simulink model "SmallFixedWingUAVupperHIL"  (R2022b)
settings: Solver=FixedStepDiscrete  StartTime=0.0  StopTime=inf  FixedStep=1/300  RelTol=1e-3
model workspace: external: MAT-File E:\RFLY\small-fixed-wing-book\fixedwing-book-rfly\ch8\code\e7-4\hitl\desire.mat (data not in the file)
values from neighbouring files (symbols this model uses):
  ctrlpoints = [xd'-xd(1);yd'-yd(1)]    [bspline.m]
  env = struct    [InitDatactrl.m]
  knots = [t1, t2, t3]    [bspline.m]
  pp = 3    [bspline.m]
  uav = struct    [InitDatactrl.m]
undefined symbols (not defined in the file or in its folder): DiscIntNeverNeededParam, RGBLED_COLOR_ENUM, RGBLED_MODE_ENUM
libraries: simulink x10, pixhawk_slib_sensors_actuators x6, pixhawk_slib_uORB_RW x5
(part 2 of 2)

== matlab function SmallFixedWingUAVupperHIL/Command/MATLAB Function8 ==
  data: n input; C output; t input; P input; U input
function C = bspline_deboor(n,t,P,U)
%     validateattributes(n, {'numeric'}, {'positive','integer','scalar'});
    d = n;  % B-spline polynomial degree (1 for linear, 2 for quadratic, etc.)
%     validateattributes(t, {'numeric'}, {'real','vector'});
%     assert(all( t(2:end)-t(1:end-1) >= 0 ), 'bspline:deboor:InvalidArgumentValue', ...
%         'Knot vector values should be nondecreasing.');
%     validateattributes(P, {'numeric'}, {'real','2d'});
%     
%     if nargin < 4
%         U = linspace(t(d+1), t(end-d), 10*size(P,2));  % allocate points uniformly
%     elseif isscalar(U) && U > 1
%         validateattributes(U, {'numeric'}, {'positive','integer','scalar'});
%         U = linspace(t(d+1), t(end-d), U);  % allocate points uniformly
%     else
%         validateattributes(U, {'numeric'}, {'real','vector'});
%         assert(all( U >= t(d+1) & U <= t(end-d) ), 'bspline:deboor:InvalidArgumentValue', ...
%             'Value outside permitted knot vector value range.');
%     end
    
    m = size(P,1);  % dimension of control points
    t = t(:).';     % knot sequence
    U = U(:);
    S = sum(bsxfun(@eq, U, t), 2);  % multiplicity of u in t (0 <= s <= d+1)
    I = bspline_deboor_interval(U,t);
    if I>length(t)-d-1
       I=length(t)-d-1;
    end
    if I == -1
        I = length(t)-d-1;
    end
    Pk = zeros(m,d+40,d+40);
    a = zeros(d+40,d+40);
    
    C = zeros(size(P,1), numel(U));
    for j = 1 : numel(U)
        u = U(j);
        s = S(j);
        ix = I(j);
        Pk(:) = 0;
        a(:) = 0;
    
        % identify d+1 relevant control points
%         Pk(:, (ix-d):(ix-s), 1) = P(:, (ix-d):(ix-s));
        h = d - s;
        if h > 0 
            Pk(:, (ix-d):(ix-s), 1) = P(:, (ix-d):(ix-s));
        end
        if h > 0
            % de Boor recursion formula
            for r = 1 : h
                q = ix-1;
                for i = (q-d+r) : (q-s)
                    a(i+1,r+1) = (u-t(i+1)) / (t(i+d-r+1+1)-t(i+1));
                    Pk(:,i+1,r+1) = (1-a(i+1,r+1)) * Pk(:,i,r) + a(i+1,r+1) * Pk(:,i+1,r);
                end
            end
            C(:,j) = Pk(:,ix-s,d-s+1);  % extract value from triangular computation scheme
        elseif ix == numel(t)  % last control point is a special case
            C(:,j) = P(:,end);
        else
            C(:,j) = P(:,ix-d);
        end
    end
end

function ix = bspline_deboor_interval(u,t)
% Index of knot in knot sequence not less than the value of u.
% If knot has multiplicity greater than 1, the highest index is returned.
    for i = 1:length(t)
        if t(i)>u
            ix = i;
            return
        end
    end
    ix = -1;
end

% function ix = bspline_deboor_interval(u,t)
% % Index of knot in knot sequence not less than the value of u.
% % If knot has multiplicity greater than 1, the highest index is returned.
% 
% i = bsxfun(@ge, u, t) & bsxfun(@lt, u, [t(2:end) 2*t(end)]);  % indicator of knot interval in which u is
% [row,col] = find(i);
% [row,ind] = sort(row);  % restore original order of data points
% ix = col(ind);
% end

== matlab function SmallFixedWingUAVupperHIL/Command/MATLAB Function9 ==
  data: p output; order input; dknots output; knots input; ctrl input; dctrl output
function [p, dknots, dctrl] = bspline_deriv(order, knots, ctrl)
    p = order;
    tmp = size(ctrl);
    n = tmp(2)-1;
    dim = tmp(1);
    
    % derivative knots
    dknots = knots(2:max(size(knots))-1);
    
    % derivative control points
    dctrl = zeros(dim,n);
    for i = 1 : n
        dctrl(:,i) = (p / (knots(i+p+1) - knots(i+1))) * (ctrl(:,i+1) - ctrl(:,i));
    end
    p = order-1;
end

== matlab function SmallFixedWingUAVupperHIL/Command/MATLAB Function ==
  data: yaw input size=[1,1]; yawdes input; roll output size=[1,1]; g input size=[1,1]; V input size=[1,1]; rolldes input
function roll = fcn(yaw,yawdes,g,V,rolldes)
%     roll = yawrate*g*V;
    if yaw>pi
        yaw = yaw-2*pi;
    end
    yawrate = 2*(yawdes-yaw);
    roll = atan2(V.*yawrate,g);
end

== matlab function SmallFixedWingUAVupperHIL/Command/MATLAB Function3 ==
  data: av1 output; Hz output; xd input; dxd input; ddxd input; x input; dx input; yaw output; g input; roll output
function [av1,Hz,yaw,roll] = DF(xd,dxd,ddxd,x,dx,g)
    av1 = (0); 
    Hz= (0); 
    yaw= (0); 
    roll= (0); 
    xd = [xd(1);xd(2);xd(3)];
    dxd = [dxd(1);dxd(2);dxd(3)];
    ddxd = [ddxd(1);ddxd(2);ddxd(3)];
    x = [x(1);x(2);x(3)];
    dx = [dx(1);dx(2);dx(3)];
%     x1 = (xd-x)/norm(xd-x);
    r1 = zeros(3,1);
    r1 = (dxd+0.2*(xd-x))/(norm(dxd+0.2*(xd-x))+0.001);
    


    av1 = ( r1'*(1*ddxd-[0;0;g]+5*(dxd-dx)+3*(xd-x)));
     %%
%     t1 = zeros(3,1,'single');
%     t2 = zeros(3,1,'single');
%     t3 = zeros(3,1,'single');
%     t4 = zeros(3,1,'single');
%     t1(1,1) = ddxd(1,1);
%     t1(2,1) = ddxd(2,1);
%     t1(3,1) = ddxd(3,1) - single(g);
%     
%     for i = 1:3
%     t2(i,1) = single(3) * (dxd(i,1) - dx(i,1));
%     t3(i,1) = single(0.1) * (xd(i,1) - x(i,1));
% 
%     end
% 
%     for i = 1:3
%     t4(i,1) = t1(i,1) + t2(i,1) + t3(i,1);
%     end
%     av1 = single( r1'*t4);
%%

    an = (eye(3)-(r1*r1'))*((ddxd)-([0;0;g]));

    av3 = -(norm(an));
    
    Hz = (xd(3));


    r3 = (an)/((av3)+(0.001));

    r2 = cross(r3,r1);

    yaw = (atan2(r1(2),r1(1)));
    
    roll = (atan2(r2(3),r3(3)));

    if isnan(av1)
        av1=(0);
    end
    if isnan(Hz)
        Hz=(0);
    end
    if isnan(yaw)
        yaw=(0);
    end

end

== matlab function SmallFixedWingUAVupperHIL/Command/InputConditioning/deadzone0 ==
  data: u input; y output
function y = fcn(u)
%Function description:
%  Control the range of the remote control input from RCMin to RCMax,which can be obtained from QGC. And set
%  a dead zone with a dead zone size of deadZone,the output y is normalized to 0~1.
RCMin = 1100;
RCMax = 1900;
RCMid = (RCMin + RCMax)/2;
deadZoneRate = 0.05;
deadZone = deadZoneRate*(RCMax - RCMin);
k = 1/(RCMax - RCMid - deadZone);
%Limiting
if(u < RCMin)
    u = RCMin;
elseif(u > RCMax)
    u = RCMax;
end
%dead zone and normalize
 if(u > RCMid + deadZone)
    y = (u-RCMid - deadZone)*k;
 elseif(u < RCMid - deadZone)
     y = (u - RCMid + deadZone)*k;
 else
     y = 0;
 end

 end

== matlab function SmallFixedWingUAVupperHIL/Command/InputConditioning/deadzone1 ==
  data: u input; y output
function y = fcn(u)
%Function description:
%  Control the range of the remote control input from RCMin to RCMax, and set
%  a dead zone with a dead zone size of ±deadZone,the output y is
%  normalized to 0~1.You can get the RC calibration parameters in QGC.
RCMin = 1100;
RCMax = 1900;
RCMid = (RCMin + RCMax)/2;
deadZoneRate = 0.05;
deadZone = deadZoneRate*(RCMax - RCMin);
k = 1/(RCMax - RCMid - deadZone);
%Limiting
if(u < RCMin)
    u = RCMin;
elseif(u > RCMax)
    u = RCMax;
end
%dead zone and normalize
 if(u > RCMid + deadZone)
    y = (u-RCMid - deadZone)*k;
 elseif(u < RCMid - deadZone)
     y = (u - RCMid + deadZone)*k;
 else
     y = 0;
 end

 end

== matlab function SmallFixedWingUAVupperHIL/Command/InputConditioning/deadzone2 ==
  data: u input; y output
function y = fcn(u)
%Function description:
%  Control the range of the remote control input from RCMin to RCMax, and set
%  a dead zone with a dead zone size of ±deadZone,the output y is
%  normalized to 0~1.You can get the RC calibration parameters in QGC.
RCMin = 1100;
RCMax = 1900;
RCMid = (RCMin + RCMax)/2;
deadZoneRate = 0.05;
deadZone = deadZoneRate*(RCMax - RCMin);
k = 1/(RCMax - RCMid - deadZone);
%Limiting
if(u < RCMin)
    u = RCMin;
elseif(u > RCMax)
    u = RCMax;
end
%dead zone and normalize
 if(u > RCMid + deadZone)
    y = (u-RCMid - deadZone)*k;
 elseif(u < RCMid - deadZone)
     y = (u - RCMid + deadZone)*k;
 else
     y = 0;
 end

 end

== matlab function SmallFixedWingUAVupperHIL/Command/InputConditioning/deadzone3 ==
  data: u input; y output
function y = fcn(u)
%Function description:
%  Control the range of the remote control input from RCMin to RCMax, and set
%  a dead zone with a dead zone size of ±deadZone,the output y is
%  normalized to 0~1.You can get the RC calibration parameters in QGC.
RCMin = 1100;
RCMax = 1900;
RCMid = (RCMin + RCMax)/2;
deadZoneRate = 0.05;
deadZone = deadZoneRate*(RCMax - RCMin);
k = 1/(RCMax - RCMid - deadZone);
%Limiting
if(u < RCMin)
    u = RCMin;
elseif(u > RCMax)
    u = RCMax;
end
%dead zone and normalize
 if(u > RCMid + deadZone)
    y = (u-RCMid - deadZone)*k;
 elseif(u < RCMid - deadZone)
     y = (u - RCMid + deadZone)*k;
 else
     y = 0;
 end

 end
